simulink model "backups"  (R2024a)
settings: Solver=VariableStepAuto  StartTime=0.0  StopTime=10.0  RelTol=1e-3
values from neighbouring files (symbols this model uses):
  AttKd_x = inp(4,2).Var2    [SFF_Simulator_Entradas.m]
  AttKd_y = inp(5,2).Var2    [SFF_Simulator_Entradas.m]
  AttKd_z = inp(6,2).Var2    [SFF_Simulator_Entradas.m]
  AttKp_x = inp(1,2).Var2    [SFF_Simulator_Entradas.m]
  AttKp_y = inp(2,2).Var2    [SFF_Simulator_Entradas.m]
  AttKp_z = inp(3,2).Var2    [SFF_Simulator_Entradas.m]
  B = inp(8,2).Var2    [SFF_Simulator_Entradas.m]
  beta = inp(2,2).Var2    [SFF_Simulator_Entradas.m]
  Cd1 = inp(4,2).Var2    [SFF_Simulator_Entradas.m]
  cdgps = inp(1,2).Var2    [SFF_Simulator_Entradas.m]
  estrelas = inp(4,2).Var2    [SFF_Simulator_Entradas.m]
  estrelas_bias = inp(6,2).Var2    [SFF_Simulator_Entradas.m]
  estrelas_ruido = inp(5,2).Var2    [SFF_Simulator_Entradas.m]
  Fn = inp(2,2).Var2    [SFF_Simulator_Entradas.m]
  gps_bias = inp(3,2).Var2    [SFF_Simulator_Entradas.m]
  gps_ruido = inp(2,2).Var2    [SFF_Simulator_Entradas.m]
  Iw = inp(7,2).Var2    [SFF_Simulator_Entradas.m]
  Ixx = inp(7,2).Var2    [SFF_Simulator_Entradas.m]
  Iyy = inp(8,2).Var2    [SFF_Simulator_Entradas.m]
  Izz = inp(9,2).Var2    [SFF_Simulator_Entradas.m]
  Km = inp(3,2).Var2    [SFF_Simulator_Entradas.m]
  Kv = inp(9,2).Var2    [SFF_Simulator_Entradas.m]
  L1 = inp(5,2).Var2    [SFF_Simulator_Entradas.m]
  limCorrente = inp(4,2).Var2    [SFF_Simulator_Entradas.m]
  limVolt = inp(5,2).Var2    [SFF_Simulator_Entradas.m]
  m1 = inp(6,2).Var2    [SFF_Simulator_Entradas.m]
  magne = inp(10,2).Var2    [SFF_Simulator_Entradas.m]
  magne_bias = inp(12,2).Var2    [SFF_Simulator_Entradas.m]
  magne_ruido = inp(11,2).Var2    [SFF_Simulator_Entradas.m]
  man = inp(1,2).Var2    [SFF_Simulator_Entradas.m]
  OrbKd_x = inp(3,2).Var2    [SFF_Simulator_Entradas.m]
  OrbKd_y = inp(6,2).Var2    [SFF_Simulator_Entradas.m]
  OrbKd_z = inp(9,2).Var2    [SFF_Simulator_Entradas.m]
  OrbKi_x = inp(2,2).Var2    [SFF_Simulator_Entradas.m]
  OrbKi_y = inp(5,2).Var2    [SFF_Simulator_Entradas.m]
  OrbKi_z = inp(8,2).Var2    [SFF_Simulator_Entradas.m]
  OrbKp_x = inp(1,2).Var2    [SFF_Simulator_Entradas.m]
  OrbKp_y = inp(4,2).Var2    [SFF_Simulator_Entradas.m]
  OrbKp_z = inp(7,2).Var2    [SFF_Simulator_Entradas.m]
  propForcaAtivo = inp(1,2).Var2    [SFF_Simulator_Entradas.m]
  Rm = inp(6,2).Var2    [SFF_Simulator_Entradas.m]
  rodaAtivo = inp(1,2).Var2    [SFF_Simulator_Entradas.m]
  RodKi = inp(1,2).Var2    [SFF_Simulator_Entradas.m]
  sat_torquerod = inp(14,2).Var2    [SFF_Simulator_Entradas.m]
  torqrodAtivo = inp(1,2).Var2    [SFF_Simulator_Entradas.m]
undefined symbols (not defined in the file or in its folder): IAU, J2, mi, omega_E, propMomentoAtivo, Re, sat_rodareacao, WMM2020
libraries: dspsrcs4 x19, aerolibtransform2 x2, aerolibgravity2 x2, simulink x1
(part 1 of 4)
settings Model: VariantFading=off  Creator=rodri  LastModifiedBy=rodri

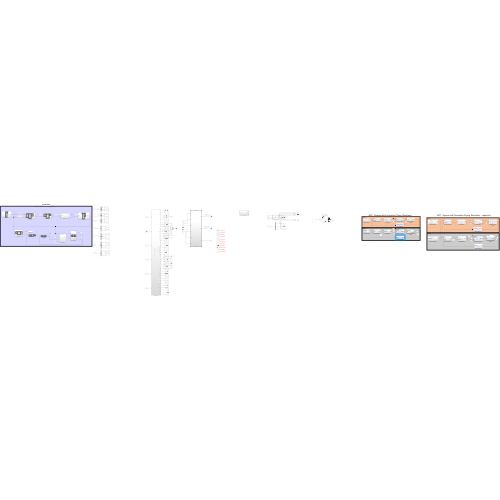
[thumbnail: Simulink's stored preview of the top-level diagram]
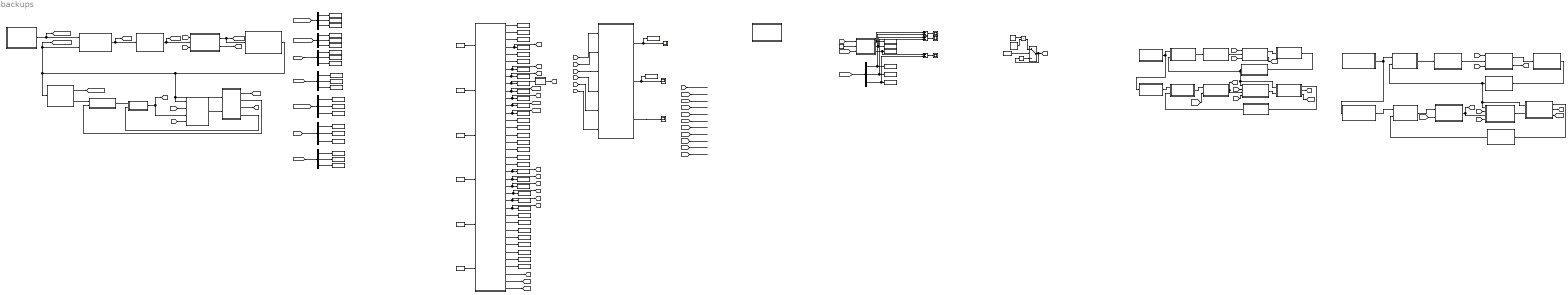
== system backups ==
  note: 13/04/2024
  note: Spacecraft Formation Flying Simulator
  note: Atitude
  note: SFF - Spacecraft Formation Flying Simulator
  note: Órbita
  note: Órbita
  note: SFF - Spacecraft Formation Flying Simulator - reduzido
  note: Atitude
  Atuadores Orbital : Subsystem
  Atuadores Orbital1 : Subsystem
  Atuadores de Atitude : Subsystem
  Atuadores de Atitude1 : Subsystem
  Bus Selector : BusSelector  OutputSignals=x_ref,y_ref,z_ref
  Bus Selector1 : BusSelector  OutputSignals=x,y,z
  Bus Selector2 : BusSelector  OutputSignals=erro_x,erro_y,erro_z
  Bus Selector3 : BusSelector  OutputSignals=phi_ref,theta_ref,psi_ref
  Bus Selector4 : BusSelector  OutputSignals=phi,theta,psi
  Constant : Constant  Value=Fn  SampleTime=-1
  Constant1 : Constant  Value=m1  SampleTime=-1
  Constant33 : Constant  Value=0
  Constant43 : Constant  Value=m1
  Constant45 : Constant  Value=0
  Constant46 : Constant  Value=0
  Constant48 : Constant  Value=Cd1
  Constant57 : Constant  Value=L1
  Controle Atitude : Subsystem
  Controle Atitude1 : Subsystem
  Controle Orbital : Subsystem
  Controle Orbital1 : Subsystem
  ControleAtitude1 : Subsystem
  Demux : Demux  Outputs=3
  Demux1 : Demux  Outputs=3
  Demux2 : Demux  Outputs=3
  Detect Decrease : simulink/Logic and Bit Operations/Detect Decrease  vinit=0.0  OutDataTypeStr=boolean
  Dinâmica Cinemática Atitude : Subsystem
  Dinâmica Cinemática Atitude1 : Subsystem
  Dinâmica Cinemática Orbital : Subsystem
  Dinâmica Cinemática Orbital1 : Subsystem
  DinâmicaCinematicaOrbital : Subsystem
  Erros Posição Orbital : Subsystem
  Erros Posição Orbital1 : Subsystem
  Erros Quatérnions : Subsystem
  Erros Quatérnions1 : Subsystem
  Guiamento Atitude : Subsystem
  Guiamento Atitude1 : Subsystem
  Guiamento Orbital : Subsystem
  Guiamento Orbital1 : Subsystem
  GuiamentoAtitude : Subsystem
  GuiamentoOrbital : Subsystem
  GuiamentoOrbital1 : Subsystem
  Memory1 : Memory  InitialCondition=Fn  InheritSampleTime=on
  Minus : Sum  Inputs=+-
  Minus1 : Sum  Inputs=+-
  Minus2 : Sum  Inputs=+-
  Product : Product
  Random Source2 : dspsrcs4/Random Source  SrcType=Uniform  MinVal=1-5/100  MaxVal=1+5/100  MeanVal=0  VarVal=1  RepMode=Not repeatable  rawSeed=1  IsInherit=off  SampTime=step_modelo  SampFrame=1  OutComplex=Real  DataType=double  SimulateUsing=Code generation
  Scope{1..6} (6 alike) : Scope
  Sensores Atitude : Subsystem
  Sensores Atitude1 : Subsystem
  Sensores Orbital : Subsystem
  Sensores Orbital1 : Subsystem
  Subsystem1 : ModelReference  ModelNameDialog=GuiamentoAtitude  ModelReferenceVersion=3.9
  Switch1 : Switch  Criteria=u2 > Threshold  SaturateOnIntegerOverflow=off  InputSameDT=off
  To Workspace : ToWorkspace  VariableName=x_ref  SaveFormat=Timeseries  SampleTime=-1
  To Workspace1 : ToWorkspace  VariableName=y_ref  SaveFormat=Timeseries  SampleTime=-1
  To Workspace10 : ToWorkspace  VariableName=uy  SaveFormat=Timeseries  SampleTime=-1
  To Workspace11 : ToWorkspace  VariableName=uz  SaveFormat=Timeseries  SampleTime=-1
  To Workspace12 : ToWorkspace  VariableName=phi_ref  SaveFormat=Timeseries  SampleTime=-1
  To Workspace13 : ToWorkspace  VariableName=theta_ref  SaveFormat=Timeseries  SampleTime=-1
  To Workspace14 : ToWorkspace  VariableName=psi_ref  SaveFormat=Timeseries  SampleTime=-1
  To Workspace15 : ToWorkspace  VariableName=phi  SaveFormat=Timeseries  SampleTime=-1
  To Workspace16 : ToWorkspace  VariableName=theta  SaveFormat=Timeseries  SampleTime=-1
  To Workspace17 : ToWorkspace  VariableName=psi  SaveFormat=Timeseries  SampleTime=-1
  To Workspace18 : ToWorkspace  VariableName=acely  SaveFormat=Timeseries  SampleTime=-1
  To Workspace19 : ToWorkspace  VariableName=acelz  SaveFormat=Timeseries  SampleTime=-1
  To Workspace2 : ToWorkspace  VariableName=z_ref  SaveFormat=Timeseries  SampleTime=-1
  To Workspace20 : ToWorkspace  VariableName=acelx  SaveFormat=Timeseries  SampleTime=-1
  To Workspace21 : ToWorkspace  VariableName=phi_ref1  SaveFormat=Timeseries  SampleTime=-1
  To Workspace22 : ToWorkspace  VariableName=theta_ref1  SaveFormat=Timeseries  SampleTime=-1
  To Workspace23 : ToWorkspace  VariableName=Fy_b_pro  SampleTime=-1
      settings: Save2DSignal=2-D array (concatenate along first dimension)
  To Workspace24 : ToWorkspace  VariableName=Fz_b_pro  SampleTime=-1
      settings: Save2DSignal=2-D array (concatenate along first dimension)
  To Workspace25 : ToWorkspace  VariableName=Fx_b_pro  SampleTime=-1
      settings: Save2DSignal=2-D array (concatenate along first dimension)
  To Workspace27 : ToWorkspace  VariableName=Fy_b_dem  SampleTime=-1
      settings: Save2DSignal=2-D array (concatenate along first dimension)
  To Workspace28 : ToWorkspace  VariableName=Fz_b_dem  SampleTime=-1
      settings: Save2DSignal=2-D array (concatenate along first dimension)
  To Workspace29 : ToWorkspace  VariableName=Fx_b_dem  SampleTime=-1
      settings: Save2DSignal=2-D array (concatenate along first dimension)
  To Workspace3 : ToWorkspace  VariableName=x  SaveFormat=Timeseries  SampleTime=-1
  To Workspace34 : ToWorkspace  VariableName=x_dotdot  SaveFormat=Timeseries  SampleTime=-1
  To Workspace35 : ToWorkspace  VariableName=y_dotdot  SaveFormat=Timeseries  SampleTime=-1
  To Workspace36 : ToWorkspace  VariableName=ohm0  SaveFormat=Timeseries  SampleTime=-1
  To Workspace37 : ToWorkspace  VariableName=omega_x  SaveFormat=Timeseries  SampleTime=-1
  To Workspace38 : ToWorkspace  VariableName=omega_z  SaveFormat=Timeseries  SampleTime=-1
  To Workspace39 : ToWorkspace  VariableName=dx0  SaveFormat=Timeseries  SampleTime=-1
  To Workspace4 : ToWorkspace  VariableName=y  SaveFormat=Timeseries  SampleTime=-1
  To Workspace40 : ToWorkspace  VariableName=dy0  SaveFormat=Timeseries  SampleTime=-1
  To Workspace41 : ToWorkspace  VariableName=dz0  SaveFormat=Timeseries  SampleTime=-1
  To Workspace47 : ToWorkspace  VariableName=delta_Dx  SaveFormat=Timeseries  SampleTime=-1
  To Workspace48 : ToWorkspace  VariableName=delta_Dy  SaveFormat=Timeseries  SampleTime=-1
  To Workspace49 : ToWorkspace  VariableName=delta_Dz  SaveFormat=Timeseries  SampleTime=-1
  To Workspace5 : ToWorkspace  VariableName=z  SaveFormat=Timeseries  SampleTime=-1
  To Workspace50 : ToWorkspace  VariableName=rho_a0  SaveFormat=Timeseries  SampleTime=-1
  To Workspace51 : ToWorkspace  VariableName=z_dotdot  SaveFormat=Timeseries  SampleTime=-1
  To Workspace52 : ToWorkspace  VariableName=x1  SaveFormat=Timeseries  SampleTime=-1
  To Workspace53 : ToWorkspace  VariableName=x_dot  SaveFormat=Timeseries  SampleTime=-1
  To Workspace54 : ToWorkspace  VariableName=y1  SaveFormat=Timeseries  SampleTime=-1
  To Workspace55 : ToWorkspace  VariableName=y_dot  SaveFormat=Timeseries  SampleTime=-1
  To Workspace56 : ToWorkspace  VariableName=z1  SaveFormat=Timeseries  SampleTime=-1
  To Workspace57 : ToWorkspace  VariableName=z_dot  SaveFormat=Timeseries  SampleTime=-1
  To Workspace58 : ToWorkspace  VariableName=rho_a1  SaveFormat=Timeseries  SampleTime=-1
  To Workspace59 : ToWorkspace  VariableName=r0_dotdot  SaveFormat=Timeseries  SampleTime=-1
  To Workspace6 : ToWorkspace  VariableName=erro_x  SaveFormat=Timeseries  SampleTime=-1
  To Workspace60 : ToWorkspace  VariableName=omega_z_dot  SaveFormat=Timeseries  SampleTime=-1
  To Workspace61 : ToWorkspace  VariableName=dx1  SaveFormat=Timeseries  SampleTime=-1
  To Workspace62 : ToWorkspace  VariableName=r0  SaveFormat=Timeseries  SampleTime=-1
  To Workspace63 : ToWorkspace  VariableName=dy1  SaveFormat=Timeseries  SampleTime=-1
  To Workspace64 : ToWorkspace  VariableName=dz1  SaveFormat=Timeseries  SampleTime=-1
  To Workspace65 : ToWorkspace  VariableName=omega_y_dot  SaveFormat=Timeseries  SampleTime=-1
  To Workspace66 : ToWorkspace  VariableName=omega_x_dot  SaveFormat=Timeseries  SampleTime=-1
  To Workspace67 : ToWorkspace  VariableName=h0  SaveFormat=Timeseries  SampleTime=-1
  To Workspace68 : ToWorkspace  VariableName=r1  SaveFormat=Timeseries  SampleTime=-1
  To Workspace69 : ToWorkspace  VariableName=r0_dot  SaveFormat=Timeseries  SampleTime=-1
  To Workspace7 : ToWorkspace  VariableName=erro_y  SaveFormat=Timeseries  SampleTime=-1
  To Workspace70 : ToWorkspace  VariableName=i0  SaveFormat=Timeseries  SampleTime=-1
  To Workspace71 : ToWorkspace  VariableName=theta0  SaveFormat=Timeseries  SampleTime=-1
  To Workspace72 : ToWorkspace  VariableName=theta0_dot  SaveFormat=Timeseries  SampleTime=-1
  To Workspace8 : ToWorkspace  VariableName=erro_z  SaveFormat=Timeseries  SampleTime=-1
  To Workspace9 : ToWorkspace  VariableName=ux  SaveFormat=Timeseries  SampleTime=-1
  atuadoresAtitude : Subsystem
  atuadoresOrbital : Subsystem
  atuadoresOrbital1 : Subsystem
  controleOrbital : Subsystem
  dinamicaCinematicaAtitude1 : Subsystem
  errosAngAtitude1 : Subsystem
  errosPosVelOrbital : Subsystem
  forçasSistCorpoSeg1 : MATLAB Function  TreatAsAtomicUnit=on
  wrapTo2Pi1 : MATLAB Function  TreatAsAtomicUnit=on
  wires:
  Bus Selector4/3 -> To Workspace17/1  "<psi>"
  Bus Selector4/2 -> To Workspace16/1  "<theta>"
  ControleAtitude1/1(Mts) -> atuadoresAtitude/3(Mts), [Mts]
  Demux/3 -> To Workspace11/1
  atuadoresAtitude/1(MtsReal) -> dinamicaCinematicaAtitude1/2(Mts)
  [atitude] -> Bus Selector4/1
  [Mts] -> atuadoresOrbital/3(Mts)
  Bus Selector4/1 -> To Workspace15/1  "<phi>"
  Bus Selector1/2 -> To Workspace4/1  "<y>"
  dinamicaCinematicaAtitude1/4(omega_rel) -> ControleAtitude1/2(omega_rel)
  [MtsProp] -> atuadoresAtitude/2(MtsProp)
  Bus Selector1/3 -> To Workspace5/1  "<z>"
  [guiamentoAtitude] -> Bus Selector3/1
  Demux1/3 -> To Workspace19/1
  Demux1/1 -> To Workspace20/1
  Bus Selector/2 -> To Workspace1/1  "<y_ref>"
  DinâmicaCinematicaOrbital/1(dinamicaCinematicaOrbital) -> atuadoresAtitude/1(dinamicaCinematicaOrbital), dinamicaCinematicaAtitude1/1(dinamicaCinematicaOrbital), errosPosVelOrbital/2(dinamicaCinematicaOrbital), [dinamicaCinematicaOrbital], GuiamentoAtitude/1(dinamicaCinematicaOrbital)
  [A_q] -> atuadoresAtitude/4(A_q)
  [acelControle] -> Demux1/1
  Bus Selector3/3 -> To Workspace14/1  "<psi_ref>"
  Bus Selector2/2 -> To Workspace7/1  "<erro_y>"
  [controleOrbital] -> Demux/1
  dinamicaCinematicaAtitude1/2(q_rel) -> errosAngAtitude1/2(q_rel)
  GuiamentoAtitude/2(q_ref) -> errosAngAtitude1/1(q_ref)
  Demux1/2 -> To Workspace18/1
  atuadoresOrbital/1(acelControle) -> [acelControle], DinâmicaCinematicaOrbital/1(controleOrbital)
  Bus Selector1/1 -> To Workspace3/1  "<x>"
  [dinamicaCinematicaOrbital] -> Bus Selector1/1
  Bus Selector2/3 -> To Workspace8/1  "<erro_z>"
  dinamicaCinematicaAtitude1/1(euler) -> [atitude]
  errosAngAtitude1/1(q_erro) -> ControleAtitude1/1(q_erro)
  [errosOrbital] -> Bus Selector2/1
  controleOrbital/1(controleOrbital) -> atuadoresOrbital/2(controleOrbital), [controleOrbital]
  Demux/1 -> To Workspace9/1
  Bus Selector2/1 -> To Workspace6/1  "<erro_x>"
  GuiamentoAtitude/1(eulerRef) -> [guiamentoAtitude]
  [A_q] -> atuadoresOrbital/1(A_q)
  Demux/2 -> To Workspace10/1
  Bus Selector3/2 -> To Workspace13/1  "<theta_ref>"
  Bus Selector/3 -> To Workspace2/1  "<z_ref>"
  errosPosVelOrbital/1(errosOrbital) -> controleOrbital/1(errosOrbital), [errosOrbital]
  Bus Selector3/1 -> To Workspace12/1  "<phi_ref>"
  Bus Selector/1 -> To Workspace/1  "<x_ref>"
  atuadoresOrbital/2(MtsProp) -> [MtsProp]
  [guiamentoOrbital] -> Bus Selector/1
  dinamicaCinematicaAtitude1/3(A_q) -> [A_q]
  GuiamentoOrbital/1(guiamentoOrbital) -> [guiamentoOrbital], errosPosVelOrbital/1(guiamentoOrbital)
  [r0] -> ?
  [theta0_dot] -> ?
  [r0_dot] -> ?
  [i0_dot] -> ?
  [omega_z] -> ?
  [omega_x] -> ?
  [omega_y] -> ?
  [ohm0] -> ?
  [ohm0_dot] -> ?
  GuiamentoOrbital1/28(r0_dotdot) -> To Workspace59/1
  GuiamentoOrbital1/30(dx1) -> To Workspace61/1
  GuiamentoOrbital1/35(i0_dot) -> [i0_dot]
  [theta0] -> ?
  GuiamentoOrbital1/21(x) -> To Workspace52/1, [x]
  GuiamentoOrbital1/15(dy0) -> To Workspace40/1
  GuiamentoOrbital1/34(omega_x_dot) -> To Workspace66/1
  GuiamentoOrbital1/11(ohm0) -> [ohm0], To Workspace36/1
  GuiamentoOrbital1/9(theta0) -> To Workspace71/1, wrapTo2Pi1/1(u)
  GuiamentoOrbital1/12(omega_x) -> To Workspace37/1, [omega_x]
  [i0] -> ?
  GuiamentoOrbital1/32(dz1) -> To Workspace64/1
  GuiamentoOrbital1/8(i0) -> [i0], To Workspace70/1
  GuiamentoOrbital1/36(ohm0_dot) -> [ohm0_dot]
  GuiamentoOrbital1/1(x_dotdot) -> To Workspace34/1
  Constant48/1 -> GuiamentoOrbital1/2(Cd1)
  GuiamentoOrbital1/22(x_dot) -> To Workspace53/1, [x_dot]
  GuiamentoOrbital1/13(omega_z) -> [omega_z], To Workspace38/1
  GuiamentoOrbital1/19(delta_Dz) -> To Workspace49/1
  GuiamentoOrbital1/20(rho_a0) -> To Workspace50/1
  Constant43/1 -> GuiamentoOrbital1/1(m1)
  GuiamentoOrbital1/10(theta0_dot) -> [theta0_dot], To Workspace72/1
  Subsystem1/2 -> Scope2/1, To Workspace22/1
  Constant33/1 -> GuiamentoOrbital1/4(ux)
  GuiamentoOrbital1/7(r0_dot) -> To Workspace69/1, [r0_dot]
  GuiamentoOrbital1/26(z_dot) -> [z_dot], To Workspace57/1
  [y_dot] -> Subsystem1/5
  GuiamentoOrbital1/3(z_dotdot) -> To Workspace51/1
  GuiamentoOrbital1/31(dy1) -> To Workspace63/1
  wrapTo2Pi1/1(y) -> [theta0]
  GuiamentoOrbital1/17(delta_Dx) -> To Workspace47/1
  GuiamentoOrbital1/2(y_dotdot) -> To Workspace35/1
  GuiamentoOrbital1/23(y) -> To Workspace54/1, [y]
  GuiamentoOrbital1/5(h0) -> To Workspace67/1
  Subsystem1/1 -> To Workspace21/1, Scope1/1
  GuiamentoOrbital1/27(rho_a1) -> To Workspace58/1
  GuiamentoOrbital1/29(omega_z_dot) -> To Workspace60/1
  GuiamentoOrbital1/6(r1) -> To Workspace68/1
  GuiamentoOrbital1/37(omega_y) -> [omega_y]
  GuiamentoOrbital1/18(delta_Dy) -> To Workspace48/1
  GuiamentoOrbital1/25(z) -> To Workspace56/1, [z]
  [x_dot] -> Subsystem1/4
  GuiamentoOrbital1/14(dx0) -> To Workspace39/1
  GuiamentoOrbital1/33(omega_y_dot) -> To Workspace65/1
  Constant45/1 -> GuiamentoOrbital1/5(uy)
  Constant46/1 -> GuiamentoOrbital1/6(uz)
  Constant57/1 -> GuiamentoOrbital1/3(l1)
  [x] -> Subsystem1/1
  [z] -> Subsystem1/3
  GuiamentoOrbital1/24(y_dot) -> To Workspace55/1, [y_dot]
  Subsystem1/3 -> Scope3/1
  [z_dot] -> Subsystem1/6
  GuiamentoOrbital1/16(dz0) -> To Workspace41/1
  GuiamentoOrbital1/4(r0) -> To Workspace62/1, [r0]
  [y] -> Subsystem1/2
  Minus2/1 -> Scope6/1
  [A_q] -> forçasSistCorpoSeg1/1(A_q)
  [controleOrbital] -> forçasSistCorpoSeg1/3(controleOrbital)
  forçasSistCorpoSeg1/1(Fx_b) -> To Workspace29/1, Minus/1
  forçasSistCorpoSeg1/2(Fy_b) -> To Workspace27/1, Minus1/1
  Demux2/3 -> To Workspace24/1, Minus2/2
  forçasSistCorpoSeg1/3(Fz_b) -> To Workspace28/1, Minus2/1
  Minus/1 -> Scope4/1
  [forcasProp] -> Demux2/1
  Constant1/1 -> forçasSistCorpoSeg1/2(m1)
  Minus1/1 -> Scope5/1
  Demux2/2 -> To Workspace23/1, Minus1/2
  Demux2/1 -> To Workspace25/1, Minus/2
  ? -> Detect Decrease/1  "PWM"
  Constant/1 -> Product/1
  Detect Decrease/1 -> Switch1/2
  Memory1/1 -> Switch1/3
  Product/1 -> Switch1/1
  Switch1/1 -> [F_real], Memory1/1
  Random Source2/1 -> Product/2
  Controle Atitude/1(Mts) -> Atuadores de Atitude/3(Mts), [Mts]
  Atuadores de Atitude/1(MtsReal) -> Dinâmica Cinemática Atitude/2(Mts)
  [omega_rel] -> Controle Atitude/2(omega_rel)
  [A_q] -> Atuadores de Atitude/4(A_q)
  [Mts] -> Atuadores Orbital/3(Mts)
  Atuadores Orbital/2(MtsProp) -> [MtsProp]
  Controle Orbital/1(conOrb) -> Atuadores Orbital/2(conOrb)
  Dinâmica Cinemática Atitude/3(omega_rel) -> [omega_rel]
  Erros Quatérnions/1(q_erro) -> Controle Atitude/1(q_erro)
  Sensores Orbital/1(dinCinOrbOut) -> Dinâmica Cinemática Atitude/1(dinCinOrb), Atuadores de Atitude/1(dinCinOrb), Erros Posição Orbital/2(dinCinOrb)
  Guiamento Orbital/1(guiOrb) -> Guiamento Atitude/1(dinCinOrb), Erros Posição Orbital/1(guiOrb)
  Dinâmica Cinemática Atitude/1(q_rel) -> Sensores Atitude/1(qRelIn)
  Dinâmica Cinemática Atitude/2(A_q) -> [A_q]
  Dinâmica Cinemática Orbital/1(dinCinOrb) -> Sensores Orbital/1(dinCinOrbIn)
  [A_q] -> Atuadores Orbital/1(A_q)
  Guiamento Atitude/1(q_ref) -> Erros Quatérnions/1(q_ref)
  Erros Posição Orbital/1(errOrb) -> Controle Orbital/1(errOrb)
  [MtsProp] -> Atuadores de Atitude/2(MtsProp)
  Atuadores Orbital/1(aceCon) -> Dinâmica Cinemática Orbital/1(conOrb)
  Sensores Atitude/1(qRelOut) -> Erros Quatérnions/2(q_rel)
  Sensores Orbital1/1(dinCinOrbSen) -> Dinâmica Cinemática Atitude1/1(dinCinOrb), Atuadores de Atitude1/1(dinCinOrb), Erros Posição Orbital1/2(dinCinOrb)
  Erros Posição Orbital1/1(errOrb) -> Controle Orbital1/1(errOrb)
  Guiamento Orbital1/1(guiOrb) -> Guiamento Atitude1/1(dinCinOrb), Erros Posição Orbital1/1(guiOrb)
  Dinâmica Cinemática Atitude1/1(q_rel) -> Sensores Atitude1/1(qRel)
  Sensores Atitude1/1(qRelSen) -> Erros Quatérnions1/2(q_rel)
  Atuadores Orbital1/1(aceCon) -> Dinâmica Cinemática Orbital1/1(conOrb)
  [A_q] -> Atuadores Orbital1/1(A_q)
  Dinâmica Cinemática Atitude1/3(omega_rel) -> [omega_rel]
  [omega_rel] -> Controle Atitude1/2(omega_rel)
  Atuadores Orbital1/2(MtsProp) -> [MtsProp]
  Erros Quatérnions1/1(q_erro) -> Controle Atitude1/1(q_erro)
  Dinâmica Cinemática Orbital1/1(dinCinOrb) -> Sensores Orbital1/1(dinCinOrb)
  [A_q] -> Atuadores de Atitude1/4(A_q)
  Controle Atitude1/1(Mts) -> Atuadores de Atitude1/3(Mts), [Mts]
  Atuadores de Atitude1/1(MtsReal) -> Dinâmica Cinemática Atitude1/2(Mts)
  Dinâmica Cinemática Atitude1/2(A_q) -> [A_q]
  Controle Orbital1/1(conOrb) -> Atuadores Orbital1/2(conOrb)
  Guiamento Atitude1/1(q_ref) -> Erros Quatérnions1/1(q_ref)
  [Mts] -> Atuadores Orbital1/3(Mts)
  [MtsProp] -> Atuadores de Atitude1/2(MtsProp)

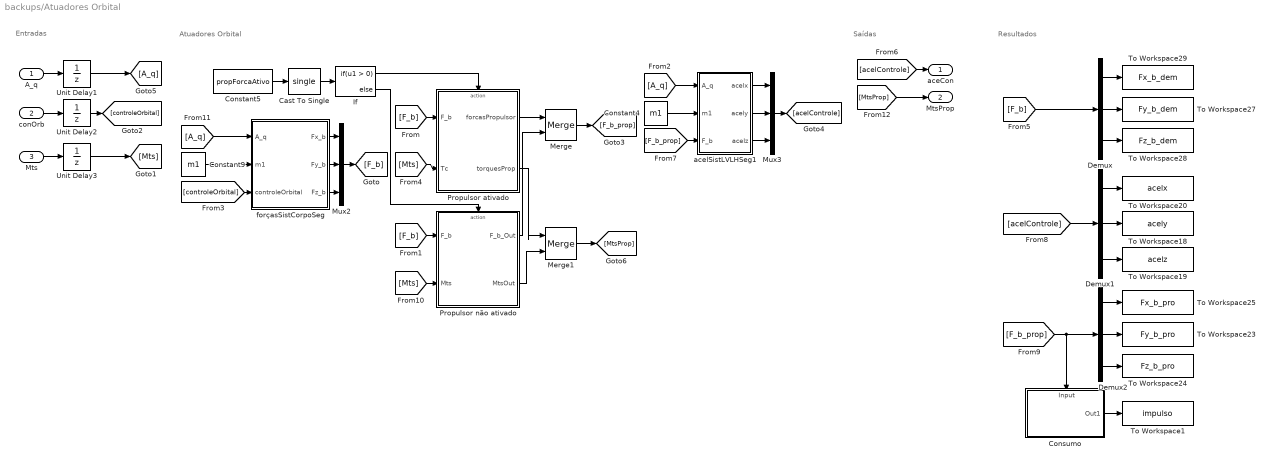
== system backups/Atuadores Orbital ==
  note: Resultados
  note: Entradas
  note: Saídas
  note: Atuadores Orbital
  A_q : Inport
  conOrb : Inport  Port=2
  Mts : Inport  Port=3
  Cast To Single : DataTypeConversion  OutDataTypeStr=single  SaturateOnIntegerOverflow=off  RndMeth=Floor
  Constant4 : Constant  Value=m1  SampleTime=-1
  Constant5 : Constant  Value=propForcaAtivo  SampleTime=-1
  Constant9 : Constant  Value=m1  SampleTime=-1
  Consumo : Subsystem
      settings: PortSchema="{\"entries\":[{\"content\":{\"sides\":[{\"content\":{},\"type\":\"ConnectorPlacement.EquallySpacedRectSide\",\"uuid\":\"7adfb598-cfd3-455e-a32c-0f282c9a4562\"},{\"content\":{\"connectorIds\":[\"Out1\"],\"side\":\"RIGHT\"},\"type\":\"ConnectorPlacement.EquallySpacedRectSide\",\"uuid\":\"983f0880-1b1d-4863-83b8-6f46272dfc63\"},{\"content\":{\"connectorIds\":[\"In1\"],\"side\":\"TOP\"},\"type\":\"ConnectorPlacement.EquallySpacedRectSide\",\"uuid\":\"1e4b7baa-07be-492c-ad2b-c1f0c72f4a8d\"}]},\"type\":\"ConnectorPlacement.EquallySpacedConnector\",\"uuid\":\"1ca021a5-bfd9-4f0e-bb93-1261a452b994\"}],\"packageUris\":[\"http://schema.mathworks.com/mf0/Connector/R2020b\"],\"version\":\"1.0\"}"
  Demux : Demux  Outputs=3
  Demux1 : Demux  Outputs=3
  Demux2 : Demux  Outputs=3
  If : If
  Merge : Merge
  Merge1 : Merge
  Mux2 : Mux  Inputs=3
  Mux3 : Mux  Inputs=3
  Propulsor ativado : Subsystem  TreatAsAtomicUnit=on
  Propulsor não ativado : Subsystem  TreatAsAtomicUnit=on
  To Workspace1 : ToWorkspace  VariableName=impulso  SampleTime=-1
      settings: Save2DSignal=2-D array (concatenate along first dimension)
  To Workspace18 : ToWorkspace  VariableName=acely  SampleTime=-1
      settings: Save2DSignal=2-D array (concatenate along first dimension)
  To Workspace19 : ToWorkspace  VariableName=acelz  SampleTime=-1
      settings: Save2DSignal=2-D array (concatenate along first dimension)
  To Workspace20 : ToWorkspace  VariableName=acelx  SampleTime=-1
      settings: Save2DSignal=2-D array (concatenate along first dimension)
  To Workspace23 : ToWorkspace  VariableName=Fy_b_pro  SampleTime=-1
      settings: Save2DSignal=2-D array (concatenate along first dimension)
  To Workspace24 : ToWorkspace  VariableName=Fz_b_pro  SampleTime=-1
      settings: Save2DSignal=2-D array (concatenate along first dimension)
  To Workspace25 : ToWorkspace  VariableName=Fx_b_pro  SampleTime=-1
      settings: Save2DSignal=2-D array (concatenate along first dimension)
  To Workspace27 : ToWorkspace  VariableName=Fy_b_dem  SampleTime=-1
      settings: Save2DSignal=2-D array (concatenate along first dimension)
  To Workspace28 : ToWorkspace  VariableName=Fz_b_dem  SampleTime=-1
      settings: Save2DSignal=2-D array (concatenate along first dimension)
  To Workspace29 : ToWorkspace  VariableName=Fx_b_dem  SampleTime=-1
      settings: Save2DSignal=2-D array (concatenate along first dimension)
  Unit Delay1 : UnitDelay  SampleTime=-1  HasFrameUpgradeWarning=on
  Unit Delay2 : UnitDelay  SampleTime=-1  HasFrameUpgradeWarning=on
  Unit Delay3 : UnitDelay  SampleTime=-1  HasFrameUpgradeWarning=on
  acelSistLVLHSeg1 : MATLAB Function  TreatAsAtomicUnit=on
  forçasSistCorpoSeg : MATLAB Function  TreatAsAtomicUnit=on
  aceCon : Outport
  MtsProp : Outport  Port=2
  wires:
  Demux1/3 -> To Workspace19/1
  Demux1/1 -> To Workspace20/1
  Demux1/2 -> To Workspace18/1
  [acelControle] -> Demux1/1
  Consumo/1(Out1) -> To Workspace1/1
  Demux/1 -> To Workspace29/1
  Demux/2 -> To Workspace27/1
  Demux/3 -> To Workspace28/1
  [F_b] -> Demux/1
  Demux2/1 -> To Workspace25/1
  [F_b_prop] -> Demux2/1, Consumo/1(Input)
  Demux2/2 -> To Workspace23/1
  Demux2/3 -> To Workspace24/1
  [A_q] -> acelSistLVLHSeg1/1(A_q)
  [acelControle] -> aceCon/1
  [F_b_prop] -> acelSistLVLHSeg1/3(F_b)
  [MtsProp] -> MtsProp/1
  Constant4/1 -> acelSistLVLHSeg1/2(m1)
  Propulsor ativado/2(torquesProp) -> Merge1/1
  Merge/1 -> [F_b_prop]
  forçasSistCorpoSeg/3(Fz_b) -> Mux2/3
  Unit Delay1/1 -> [A_q]
  Merge1/1 -> [MtsProp]
  forçasSistCorpoSeg/1(Fx_b) -> Mux2/1
  If/2 -> Propulsor não ativado/Action
  If/1 -> Propulsor ativado/Action
  Unit Delay2/1 -> [controleOrbital]
  [Mts] -> Propulsor não ativado/2(Mts)
  [A_q] -> forçasSistCorpoSeg/1(A_q)
  Constant9/1 -> forçasSistCorpoSeg/2(m1)
  [controleOrbital] -> forçasSistCorpoSeg/3(controleOrbital)
  [Mts] -> Propulsor ativado/2(Tc)
  acelSistLVLHSeg1/1(acelx) -> Mux3/1
  Mux3/1 -> [acelControle]
  acelSistLVLHSeg1/3(acelz) -> Mux3/3
  acelSistLVLHSeg1/2(acely) -> Mux3/2
  forçasSistCorpoSeg/2(Fy_b) -> Mux2/2
  Propulsor ativado/1(forcasPropulsor) -> Merge/1
  Cast To Single/1 -> If/1
  Mux2/1 -> [F_b]
  Mts/1 -> Unit Delay3/1
  [F_b] -> Propulsor não ativado/1(F_b)
  conOrb/1 -> Unit Delay2/1
  Propulsor não ativado/1(F_b_Out) -> Merge/2
  Unit Delay3/1 -> [Mts]
  Constant5/1 -> Cast To Single/1
  [F_b] -> Propulsor ativado/1(F_b)
  Propulsor não ativado/2(MtsOut) -> Merge1/2
  A_q/1 -> Unit Delay1/1

== system backups/Atuadores Orbital1 ==
  note: Saídas
  note: Resultados
  note: Atuadores Orbital
  note: Entradas
  A_q : Inport
  conOrb : Inport  Port=2
  Mts : Inport  Port=3
  Cast To Single : DataTypeConversion  OutDataTypeStr=single  SaturateOnIntegerOverflow=off  RndMeth=Floor
  Constant4 : Constant  Value=m1  SampleTime=-1
  Constant5 : Constant  Value=propForcaAtivo  SampleTime=-1
  Constant9 : Constant  Value=m1  SampleTime=-1
  Consumo : Subsystem
      settings: PortSchema="{\"entries\":[{\"content\":{\"sides\":[{\"content\":{},\"type\":\"ConnectorPlacement.EquallySpacedRectSide\",\"uuid\":\"7adfb598-cfd3-455e-a32c-0f282c9a4562\"},{\"content\":{\"connectorIds\":[\"Out1\"],\"side\":\"RIGHT\"},\"type\":\"ConnectorPlacement.EquallySpacedRectSide\",\"uuid\":\"983f0880-1b1d-4863-83b8-6f46272dfc63\"},{\"content\":{\"connectorIds\":[\"In1\"],\"side\":\"TOP\"},\"type\":\"ConnectorPlacement.EquallySpacedRectSide\",\"uuid\":\"1e4b7baa-07be-492c-ad2b-c1f0c72f4a8d\"}]},\"type\":\"ConnectorPlacement.EquallySpacedConnector\",\"uuid\":\"1ca021a5-bfd9-4f0e-bb93-1261a452b994\"}],\"packageUris\":[\"http://schema.mathworks.com/mf0/Connector/R2020b\"],\"version\":\"1.0\"}"
  If : If
  Merge : Merge
  Merge1 : Merge
  Mux2 : Mux  Inputs=3
  Mux3 : Mux  Inputs=3
  Propulsor ativado : Subsystem  TreatAsAtomicUnit=on
  Propulsor não ativado : Subsystem  TreatAsAtomicUnit=on
  To Workspace1 : ToWorkspace  VariableName=impulso  SampleTime=-1
      settings: Save2DSignal=2-D array (concatenate along first dimension)
  Unit Delay1 : UnitDelay  SampleTime=-1  HasFrameUpgradeWarning=on
  Unit Delay2 : UnitDelay  SampleTime=-1  HasFrameUpgradeWarning=on
  Unit Delay3 : UnitDelay  SampleTime=-1  HasFrameUpgradeWarning=on
  acelSistLVLHSeg1 : MATLAB Function  TreatAsAtomicUnit=on
  forçasSistCorpoSeg : MATLAB Function  TreatAsAtomicUnit=on
  aceCon : Outport
  MtsProp : Outport  Port=2
  wires:
  A_q/1 -> Unit Delay1/1
  conOrb/1 -> Unit Delay2/1
  Mts/1 -> Unit Delay3/1
  Constant5/1 -> Cast To Single/1
  Cast To Single/1 -> If/1
  If/1 -> Propulsor ativado/Action
  [Mts] -> Propulsor não ativado/2(Mts)
  [F_b] -> Propulsor não ativado/1(F_b)
  Propulsor não ativado/1(F_b_Out) -> Merge/2
  Propulsor ativado/1(forcasPropulsor) -> Merge/1
  Propulsor não ativado/2(MtsOut) -> Merge1/2
  Propulsor ativado/2(torquesProp) -> Merge1/1
  [F_b] -> Propulsor ativado/1(F_b)
  If/2 -> Propulsor não ativado/Action
  Unit Delay1/1 -> [A_q]
  Unit Delay2/1 -> [controleOrbital]
  Unit Delay3/1 -> [Mts]
  Mux2/1 -> [F_b]
  [A_q] -> forçasSistCorpoSeg/1(A_q)
  forçasSistCorpoSeg/3(Fz_b) -> Mux2/3
  Constant9/1 -> forçasSistCorpoSeg/2(m1)
  [controleOrbital] -> forçasSistCorpoSeg/3(controleOrbital)
  forçasSistCorpoSeg/2(Fy_b) -> Mux2/2
  forçasSistCorpoSeg/1(Fx_b) -> Mux2/1
  [Mts] -> Propulsor ativado/2(Tc)
  acelSistLVLHSeg1/3(acelz) -> Mux3/3
  Constant4/1 -> acelSistLVLHSeg1/2(m1)
  acelSistLVLHSeg1/1(acelx) -> Mux3/1
  [F_b_prop] -> acelSistLVLHSeg1/3(F_b)
  acelSistLVLHSeg1/2(acely) -> Mux3/2
  Mux3/1 -> [acelControle]
  [A_q] -> acelSistLVLHSeg1/1(A_q)
  Consumo/1(Out1) -> To Workspace1/1
  [acelControle] -> aceCon/1
  Merge/1 -> [F_b_prop]
  [F_b_prop] -> Consumo/1(Input)
  Merge1/1 -> [MtsProp]
  [MtsProp] -> MtsProp/1

== system backups/Atuadores de Atitude ==
  note: Entradas
  note: Atuadores Atitude
  note: Saídas
  dinCinOrb : Inport
  MtsProp : Inport  Port=2
  Mts : Inport  Port=3
  A_q : Inport  Port=4
  Atuador atitude ativado : Subsystem  TreatAsAtomicUnit=on
  Atuador atitude desativado : Subsystem  TreatAsAtomicUnit=on
  Cast To Single : DataTypeConversion  OutDataTypeStr=single  SaturateOnIntegerOverflow=off  RndMeth=Floor
  Constant4 : Constant  Value=rodaAtivo  SampleTime=-1
  Constant5 : Constant  Value=propForcaAtivo  SampleTime=-1
  Constant9 : Constant  Value=torqrodAtivo  SampleTime=-1
  If : If
  Logical Operator : Logic  Operator=OR  Inputs=3  AllPortsSameDT=off  OutDataTypeStr=boolean
  Merge : Merge
  MtsReal : Outport
  wires:
  Mts/1 -> [Mts]
  dinCinOrb/1 -> [dinCinOrb]
  MtsProp/1 -> [MtsProp]
  Merge/1 -> [MtsReal]
  If/1 -> Atuador atitude ativado/Action
  If/2 -> Atuador atitude desativado/Action
  Atuador atitude ativado/1(MtsReal) -> Merge/1
  Atuador atitude desativado/1(Out1) -> Merge/2
  [Mts] -> Atuador atitude desativado/1(In1)
  [MtsProp] -> Atuador atitude ativado/1(MtsProp)
  [Mts] -> Atuador atitude ativado/2(Mts)
  [dinCinOrb] -> Atuador atitude ativado/3(dinCinOrb)
  [A_q] -> Atuador atitude ativado/4(A_q)
  A_q/1 -> [A_q]
  [MtsReal] -> MtsReal/1
  Constant5/1 -> Logical Operator/1
  Logical Operator/1 -> Cast To Single/1
  Cast To Single/1 -> If/1
  Constant4/1 -> Logical Operator/2
  Constant9/1 -> Logical Operator/3

== system backups/Atuadores de Atitude1 ==
  note: Entradas
  note: Atuadores Atitude
  note: Saídas
  dinCinOrb : Inport
  MtsProp : Inport  Port=2
  Mts : Inport  Port=3
  A_q : Inport  Port=4
  Atuador atitude ativado : Subsystem  TreatAsAtomicUnit=on
  Atuador atitude desativado : Subsystem  TreatAsAtomicUnit=on
  Cast To Single : DataTypeConversion  OutDataTypeStr=single  SaturateOnIntegerOverflow=off  RndMeth=Floor
  Constant4 : Constant  Value=rodaAtivo  SampleTime=-1
  Constant5 : Constant  Value=propForcaAtivo  SampleTime=-1
  Constant9 : Constant  Value=torqrodAtivo  SampleTime=-1
  If : If
  Logical Operator : Logic  Operator=OR  Inputs=3  AllPortsSameDT=off  OutDataTypeStr=boolean
  Merge : Merge
  MtsReal : Outport
  wires:
  Mts/1 -> [Mts]
  dinCinOrb/1 -> [dinCinOrb]
  MtsProp/1 -> [MtsProp]
  Merge/1 -> [MtsReal]
  Logical Operator/1 -> Cast To Single/1
  Constant5/1 -> Logical Operator/1
  Constant4/1 -> Logical Operator/2
  Constant9/1 -> Logical Operator/3
  Cast To Single/1 -> If/1
  If/1 -> Atuador atitude ativado/Action
  If/2 -> Atuador atitude desativado/Action
  Atuador atitude ativado/1(MtsReal) -> Merge/1
  Atuador atitude desativado/1(Out1) -> Merge/2
  [Mts] -> Atuador atitude desativado/1(In1)
  [MtsProp] -> Atuador atitude ativado/1(MtsProp)
  [Mts] -> Atuador atitude ativado/2(Mts)
  [dinCinOrb] -> Atuador atitude ativado/3(dinCinOrb)
  [A_q] -> Atuador atitude ativado/4(A_q)
  A_q/1 -> [A_q]
  [MtsReal] -> MtsReal/1

== system backups/Controle Atitude ==
  note: Entradas
  note: Controle de Atitude
  note: Saídas
  note: Resultados
  q_erro : Inport
  omega_rel : Inport  Port=2
  Demux : Demux
  Demux1 : Demux  Outputs=3
  Demux3 : Demux  Outputs=3
  Gain1 : Gain  Gain=-1
  Kd1 : Gain  Gain=[AttKd_x AttKd_y AttKd_z]'
  Kp1 : Gain  Gain=[AttKp_x AttKp_y AttKp_z]'
  Mux : Mux  Inputs=3
  Sum3 : Sum  Inputs=|++
  Terminator : Terminator
  To Workspace24 : ToWorkspace  VariableName=Mts_x  SampleTime=-1
      settings: Save2DSignal=2-D array (concatenate along first dimension)
  To Workspace25 : ToWorkspace  VariableName=Mts_y  SampleTime=-1
      settings: Save2DSignal=2-D array (concatenate along first dimension)
  To Workspace26 : ToWorkspace  VariableName=Mts_z  SampleTime=-1
      settings: Save2DSignal=2-D array (concatenate along first dimension)
  Unit Delay : UnitDelay  SampleTime=-1  HasFrameUpgradeWarning=on
  Unit Delay1 : UnitDelay  SampleTime=-1  HasFrameUpgradeWarning=on
  Vector Concatenate1 : Concatenate  NumInputs=3  Mode=Multidimensional array
  Mts : Outport
  wires:
  [q_erro] -> Demux/1
  Mux/1 -> Kp1/1
  Demux/1 -> Mux/1
  Demux/2 -> Mux/2
  Demux/3 -> Mux/3
  Demux/4 -> Terminator/1
  [omega_rel] -> Kd1/1
  Kd1/1 -> Sum3/2
  Sum3/1 -> Demux1/1
  Demux1/1 -> Vector Concatenate1/1
  Demux1/2 -> Vector Concatenate1/2
  Demux1/3 -> Vector Concatenate1/3
  q_erro/1 -> Unit Delay/1
  omega_rel/1 -> Unit Delay1/1
  [Mts] -> Mts/1
  Vector Concatenate1/1 -> Gain1/1
  Gain1/1 -> [Mts]
  Kp1/1 -> Sum3/1
  Demux3/3 -> To Workspace26/1
  Demux3/2 -> To Workspace25/1
  Demux3/1 -> To Workspace24/1
  [Mts] -> Demux3/1
  Unit Delay/1 -> [q_erro]
  Unit Delay1/1 -> [omega_rel]

== system backups/Controle Atitude1 ==
  note: Entradas
  note: Controle de Atitude
  note: Saídas
  note: Resultados
  q_erro : Inport
  omega_rel : Inport  Port=2
  Demux : Demux
  Demux1 : Demux  Outputs=3
  Gain1 : Gain  Gain=-1
  Kd1 : Gain  Gain=[AttKd_x AttKd_y AttKd_z]'
  Kp1 : Gain  Gain=[AttKp_x AttKp_y AttKp_z]'
  Mux : Mux  Inputs=3
  Sum3 : Sum  Inputs=|++
  Terminator : Terminator
  Unit Delay : UnitDelay  SampleTime=-1  HasFrameUpgradeWarning=on
  Unit Delay1 : UnitDelay  SampleTime=-1  HasFrameUpgradeWarning=on
  Vector Concatenate1 : Concatenate  NumInputs=3  Mode=Multidimensional array
  Mts : Outport
  wires:
  [q_erro] -> Demux/1
  Mux/1 -> Kp1/1
  Demux/1 -> Mux/1
  Demux/2 -> Mux/2
  Demux/3 -> Mux/3
  Demux/4 -> Terminator/1
  [omega_rel] -> Kd1/1
  Kd1/1 -> Sum3/2
  Sum3/1 -> Demux1/1
  Demux1/1 -> Vector Concatenate1/1
  Demux1/2 -> Vector Concatenate1/2
  Demux1/3 -> Vector Concatenate1/3
  q_erro/1 -> Unit Delay/1
  omega_rel/1 -> Unit Delay1/1
  [Mts] -> Mts/1
  Vector Concatenate1/1 -> Gain1/1
  Gain1/1 -> [Mts]
  Kp1/1 -> Sum3/1
  Unit Delay/1 -> [q_erro]
  Unit Delay1/1 -> [omega_rel]

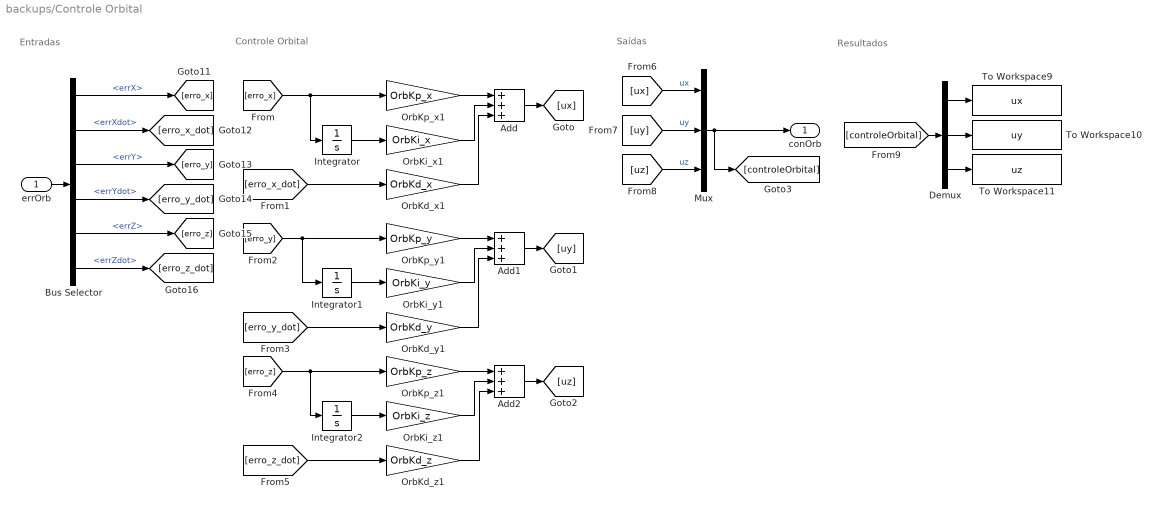
== system backups/Controle Orbital ==
  note: Entradas
  note: Controle Orbital
  note: Saídas
  note: Resultados
  errOrb : Inport
  Add : Sum  Inputs=+++
  Add1 : Sum  Inputs=+++
  Add2 : Sum  Inputs=+++
  Bus Selector : BusSelector  OutputSignals=errX,errXdot,errY,errYdot,errZ,errZdot
  Demux : Demux  Outputs=3
  Integrator : Integrator
  Integrator1 : Integrator
  Integrator2 : Integrator
  Mux : Mux  Inputs=3
  OrbKd_x1 : Gain  Gain=OrbKd_x
  OrbKd_y1 : Gain  Gain=OrbKd_y
  OrbKd_z1 : Gain  Gain=OrbKd_z
  OrbKi_x1 : Gain  Gain=OrbKi_x
  OrbKi_y1 : Gain  Gain=OrbKi_y
  OrbKi_z1 : Gain  Gain=OrbKi_z
  OrbKp_x1 : Gain  Gain=OrbKp_x
  OrbKp_y1 : Gain  Gain=OrbKp_y
  OrbKp_z1 : Gain  Gain=OrbKp_z
  To Workspace10 : ToWorkspace  VariableName=uy  SampleTime=-1
      settings: Save2DSignal=2-D array (concatenate along first dimension)
  To Workspace11 : ToWorkspace  VariableName=uz  SampleTime=-1
      settings: Save2DSignal=2-D array (concatenate along first dimension)
  To Workspace9 : ToWorkspace  VariableName=ux  SampleTime=-1
      settings: Save2DSignal=2-D array (concatenate along first dimension)
  conOrb : Outport
  wires:
  Add/1 -> [ux]
  Add1/1 -> [uy]
  Add2/1 -> [uz]
  Bus Selector/6 -> [erro_z_dot]  "<errZdot>"
  Bus Selector/4 -> [erro_y_dot]  "<errYdot>"
  Bus Selector/3 -> [erro_y]  "<errY>"
  Bus Selector/1 -> [erro_x]  "<errX>"
  Bus Selector/5 -> [erro_z]  "<errZ>"
  Bus Selector/2 -> [erro_x_dot]  "<errXdot>"
  errOrb/1 -> Bus Selector/1
  [ux] -> Mux/1  "ux"
  [uy] -> Mux/2  "uy"
  [uz] -> Mux/3  "uz"
  [erro_x_dot] -> OrbKd_x1/1
  Integrator1/1 -> OrbKi_y1/1
  Integrator2/1 -> OrbKi_z1/1
  [erro_y] -> OrbKp_y1/1, Integrator1/1
  OrbKi_z1/1 -> Add2/2
  OrbKi_x1/1 -> Add/2
  OrbKp_x1/1 -> Add/1
  OrbKd_x1/1 -> Add/3
  [erro_x] -> OrbKp_x1/1, Integrator/1
  OrbKi_y1/1 -> Add1/2
  OrbKp_y1/1 -> Add1/1
  Integrator/1 -> OrbKi_x1/1
  OrbKd_y1/1 -> Add1/3
  [erro_z_dot] -> OrbKd_z1/1
  OrbKd_z1/1 -> Add2/3
  [erro_y_dot] -> OrbKd_y1/1
  [erro_z] -> OrbKp_z1/1, Integrator2/1
  OrbKp_z1/1 -> Add2/1
  Mux/1 -> conOrb/1, [controleOrbital]
  Demux/3 -> To Workspace11/1
  [controleOrbital] -> Demux/1
  Demux/1 -> To Workspace9/1
  Demux/2 -> To Workspace10/1

== system backups/Controle Orbital1 ==
  note: Entradas
  note: Controle Orbital
  note: Saídas
  note: Resultados
  errOrb : Inport
  Add : Sum  Inputs=+++
  Add1 : Sum  Inputs=+++
  Add2 : Sum  Inputs=+++
  Bus Selector : BusSelector  OutputSignals=errX,errXdot,errY,errYdot,errZ,errZdot
  Integrator : Integrator
  Integrator1 : Integrator
  Integrator2 : Integrator
  Mux : Mux  Inputs=3
  OrbKd_x1 : Gain  Gain=OrbKd_x
  OrbKd_y1 : Gain  Gain=OrbKd_y
  OrbKd_z1 : Gain  Gain=OrbKd_z
  OrbKi_x1 : Gain  Gain=OrbKi_x
  OrbKi_y1 : Gain  Gain=OrbKi_y
  OrbKi_z1 : Gain  Gain=OrbKi_z
  OrbKp_x1 : Gain  Gain=OrbKp_x
  OrbKp_y1 : Gain  Gain=OrbKp_y
  OrbKp_z1 : Gain  Gain=OrbKp_z
  conOrb : Outport
  wires:
  Add/1 -> [ux]
  Add1/1 -> [uy]
  Add2/1 -> [uz]
  Bus Selector/6 -> [erro_z_dot]  "<errZdot>"
  Bus Selector/4 -> [erro_y_dot]  "<errYdot>"
  Bus Selector/3 -> [erro_y]  "<errY>"
  Bus Selector/1 -> [erro_x]  "<errX>"
  Bus Selector/5 -> [erro_z]  "<errZ>"
  Bus Selector/2 -> [erro_x_dot]  "<errXdot>"
  errOrb/1 -> Bus Selector/1
  [ux] -> Mux/1  "ux"
  [uy] -> Mux/2  "uy"
  [uz] -> Mux/3  "uz"
  [erro_x_dot] -> OrbKd_x1/1
  Integrator1/1 -> OrbKi_y1/1
  Integrator2/1 -> OrbKi_z1/1
  [erro_y] -> OrbKp_y1/1, Integrator1/1
  OrbKi_z1/1 -> Add2/2
  OrbKi_x1/1 -> Add/2
  OrbKp_x1/1 -> Add/1
  OrbKd_x1/1 -> Add/3
  [erro_x] -> OrbKp_x1/1, Integrator/1
  OrbKi_y1/1 -> Add1/2
  OrbKp_y1/1 -> Add1/1
  Integrator/1 -> OrbKi_x1/1
  OrbKd_y1/1 -> Add1/3
  [erro_z_dot] -> OrbKd_z1/1
  OrbKd_z1/1 -> Add2/3
  [erro_y_dot] -> OrbKd_y1/1
  [erro_z] -> OrbKp_z1/1, Integrator2/1
  OrbKp_z1/1 -> Add2/1
  Mux/1 -> conOrb/1, [controleOrbital]

== system backups/ControleAtitude1 ==
  note: Entradas
  note: Planta
  note: Saídas
  q_erro : Inport
  omega_rel : Inport  Port=2
  Demux : Demux
  Demux1 : Demux  Outputs=3
  Gain1 : Gain  Gain=-1
  Kd1 : Gain  Gain=[AttKd_x AttKd_y AttKd_z]'
  Kp1 : Gain  Gain=[AttKp_x AttKp_y AttKp_z]'
  Mux : Mux  Inputs=3
  Sum3 : Sum  Inputs=|++
  Terminator : Terminator
  Vector Concatenate1 : Concatenate  NumInputs=3  Mode=Multidimensional array
  Mts : Outport
  wires:
  [q_erro] -> Demux/1
  Mux/1 -> Kp1/1
  Demux/1 -> Mux/1
  Demux/2 -> Mux/2
  Demux/3 -> Mux/3
  Demux/4 -> Terminator/1
  [omega_rel] -> Kd1/1
  Kd1/1 -> Sum3/2
  Sum3/1 -> Demux1/1
  Demux1/1 -> Vector Concatenate1/1
  Demux1/2 -> Vector Concatenate1/2
  Demux1/3 -> Vector Concatenate1/3
  q_erro/1 -> [q_erro]
  omega_rel/1 -> [omega_rel]
  [Mts] -> Mts/1
  Vector Concatenate1/1 -> Gain1/1
  Gain1/1 -> [Mts]
  Kp1/1 -> Sum3/1

== system backups/Dinâmica Cinemática Atitude ==
  note: Dinâmica e Cinemática de Atitude
  note: Saídas
  note: Entradas
  note: Resultados
  dinCinOrb : Inport
  Mts : Inport  Port=2
  Bus Creator : BusCreator  Inputs=3
  Bus Selector : BusSelector  OutputSignals=omega_x,omega_y,omega_z,omega_x_dot,omega_y_dot,omega_z_dot
  Bus Selector4 : BusSelector  OutputSignals=phi,theta,psi
  DinamicaCinematicaAtitude : ModelReference  ModelNameDialog=DinamicaCinematicaControleAtitude  ModelReferenceVersion=3.14
  MATLAB Function : MATLAB Function  TreatAsAtomicUnit=on
  To Workspace15 : ToWorkspace  VariableName=phi  SampleTime=-1
      settings: Save2DSignal=2-D array (concatenate along first dimension)
  To Workspace16 : ToWorkspace  VariableName=theta  SampleTime=-1
      settings: Save2DSignal=2-D array (concatenate along first dimension)
  To Workspace17 : ToWorkspace  VariableName=psi  SampleTime=-1
      settings: Save2DSignal=2-D array (concatenate along first dimension)
  Vector Concatenate : Concatenate  NumInputs=3  Mode=Multidimensional array
  Vector Concatenate1 : Concatenate  NumInputs=3  Mode=Multidimensional array
  q_rel : Outport
  A_q : Outport  Port=2
  omega_rel : Outport  Port=3
  wires:
  DinamicaCinematicaAtitude/1 -> [q_rel]
  DinamicaCinematicaAtitude/2 -> [A_q]
  [q_rel] -> q_rel/1
  dinCinOrb/1 -> Bus Selector/1
  [omega_i] -> DinamicaCinematicaAtitude/2
  [omega_i_dot] -> DinamicaCinematicaAtitude/3
  [Mts] -> DinamicaCinematicaAtitude/1
  Bus Selector/1 -> Vector Concatenate1/1  "<omega_x>"
  Bus Selector/3 -> Vector Concatenate1/3  "<omega_z>"
  Bus Selector/2 -> Vector Concatenate1/2  "<omega_y>"
  Vector Concatenate1/1 -> [omega_i]
  Bus Selector/4 -> Vector Concatenate/1  "<omega_x_dot>"
  Bus Selector/5 -> Vector Concatenate/2  "<omega_y_dot>"
  Bus Selector/6 -> Vector Concatenate/3  "<omega_z_dot>"
  Vector Concatenate/1 -> [omega_i_dot]
  DinamicaCinematicaAtitude/3 -> [omega_rel]
  Mts/1 -> [Mts]
  [q_rel] -> MATLAB Function/1(u)
  MATLAB Function/1(phi) -> Bus Creator/1
  MATLAB Function/2(theta) -> Bus Creator/2
  MATLAB Function/3(psi) -> Bus Creator/3
  [A_q] -> A_q/1
  [omega_rel] -> omega_rel/1
  Bus Selector4/2 -> To Workspace16/1  "<theta>"
  Bus Selector4/1 -> To Workspace15/1  "<phi>"
  [atitude] -> Bus Selector4/1
  Bus Selector4/3 -> To Workspace17/1  "<psi>"
  Bus Creator/1 -> [atitude]

== system backups/Dinâmica Cinemática Atitude1 ==
  note: Dinâmica e Cinemática de Atitude
  note: Saídas
  note: Entradas
  note: Resultados
  dinCinOrb : Inport
  Mts : Inport  Port=2
  Bus Creator : BusCreator  Inputs=3
  Bus Selector : BusSelector  OutputSignals=omega_x,omega_y,omega_z,omega_x_dot,omega_y_dot,omega_z_dot
  Bus Selector4 : BusSelector  OutputSignals=phi,theta,psi
  DinamicaCinematicaAtitude : ModelReference  ModelNameDialog=DinamicaCinematicaControleAtitude  ModelReferenceVersion=3.14
  MATLAB Function : MATLAB Function  TreatAsAtomicUnit=on
  To Workspace15 : ToWorkspace  VariableName=phi  SampleTime=-1
      settings: Save2DSignal=2-D array (concatenate along first dimension)
  To Workspace16 : ToWorkspace  VariableName=theta  SampleTime=-1
      settings: Save2DSignal=2-D array (concatenate along first dimension)
  To Workspace17 : ToWorkspace  VariableName=psi  SampleTime=-1
      settings: Save2DSignal=2-D array (concatenate along first dimension)
  Vector Concatenate : Concatenate  NumInputs=3  Mode=Multidimensional array
  Vector Concatenate1 : Concatenate  NumInputs=3  Mode=Multidimensional array
  q_rel : Outport
  A_q : Outport  Port=2
  omega_rel : Outport  Port=3
  wires:
  DinamicaCinematicaAtitude/1 -> [q_rel]
  DinamicaCinematicaAtitude/2 -> [A_q]
  [q_rel] -> q_rel/1
  dinCinOrb/1 -> Bus Selector/1
  [omega_i] -> DinamicaCinematicaAtitude/2
  [omega_i_dot] -> DinamicaCinematicaAtitude/3
  [Mts] -> DinamicaCinematicaAtitude/1
  Bus Selector/1 -> Vector Concatenate1/1  "<omega_x>"
  Bus Selector/3 -> Vector Concatenate1/3  "<omega_z>"
  Bus Selector/2 -> Vector Concatenate1/2  "<omega_y>"
  Vector Concatenate1/1 -> [omega_i]
  Bus Selector/4 -> Vector Concatenate/1  "<omega_x_dot>"
  Bus Selector/5 -> Vector Concatenate/2  "<omega_y_dot>"
  Bus Selector/6 -> Vector Concatenate/3  "<omega_z_dot>"
  Vector Concatenate/1 -> [omega_i_dot]
  DinamicaCinematicaAtitude/3 -> [omega_rel]
  Mts/1 -> [Mts]
  [q_rel] -> MATLAB Function/1(u)
  MATLAB Function/1(phi) -> Bus Creator/1
  MATLAB Function/2(theta) -> Bus Creator/2
  MATLAB Function/3(psi) -> Bus Creator/3
  [A_q] -> A_q/1
  [omega_rel] -> omega_rel/1
  Bus Selector4/2 -> To Workspace16/1  "<theta>"
  Bus Selector4/1 -> To Workspace15/1  "<phi>"
  [atitude] -> Bus Selector4/1
  Bus Selector4/3 -> To Workspace17/1  "<psi>"
  Bus Creator/1 -> [atitude]

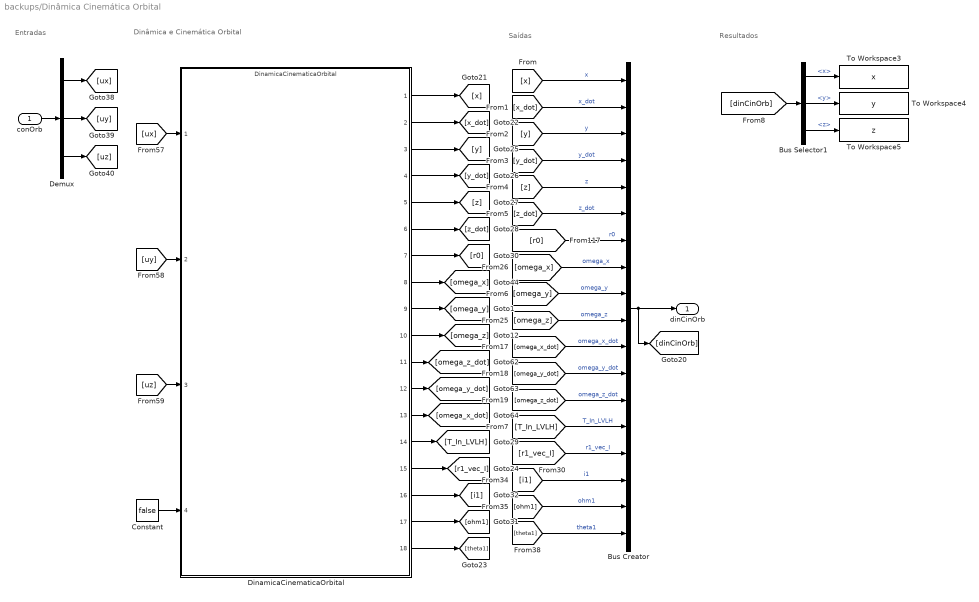
== system backups/Dinâmica Cinemática Orbital ==
  note: Entradas
  note: Saídas
  note: Dinâmica e Cinemática Orbital
  note: Resultados
  conOrb : Inport  OutDataTypeStr=double
  Bus Creator : BusCreator  Inputs=18
  Bus Selector1 : BusSelector  OutputSignals=x,y,z
  Constant : Constant  Value=false
  Demux : Demux  Outputs=3
  DinamicaCinematicaOrbital : ModelReference  ModelNameDialog=DinamicaCinematicaOrbital  ModelReferenceVersion=5.18
  To Workspace3 : ToWorkspace  VariableName=x  SampleTime=-1
      settings: Save2DSignal=2-D array (concatenate along first dimension)
  To Workspace4 : ToWorkspace  VariableName=y  SampleTime=-1
      settings: Save2DSignal=2-D array (concatenate along first dimension)
  To Workspace5 : ToWorkspace  VariableName=z  SampleTime=-1
      settings: Save2DSignal=2-D array (concatenate along first dimension)
  dinCinOrb : Outport
  wires:
  conOrb/1 -> Demux/1
  Demux/1 -> [ux]
  Demux/2 -> [uy]
  Demux/3 -> [uz]
  [ux] -> DinamicaCinematicaOrbital/1
  [uy] -> DinamicaCinematicaOrbital/2
  [uz] -> DinamicaCinematicaOrbital/3
  Constant/1 -> DinamicaCinematicaOrbital/4
  Bus Creator/1 -> dinCinOrb/1, [dinCinOrb]
  Bus Selector1/1 -> To Workspace3/1  "<x>"
  Bus Selector1/2 -> To Workspace4/1  "<y>"
  Bus Selector1/3 -> To Workspace5/1  "<z>"
  [dinCinOrb] -> Bus Selector1/1
  DinamicaCinematicaOrbital/2 -> [x_dot]
  DinamicaCinematicaOrbital/5 -> [z]
  DinamicaCinematicaOrbital/4 -> [y_dot]
  DinamicaCinematicaOrbital/6 -> [z_dot]
  DinamicaCinematicaOrbital/7 -> [r0]
  DinamicaCinematicaOrbital/3 -> [y]
  DinamicaCinematicaOrbital/1 -> [x]
  DinamicaCinematicaOrbital/8 -> [omega_x]
  DinamicaCinematicaOrbital/10 -> [omega_z]
  DinamicaCinematicaOrbital/11 -> [omega_z_dot]
  DinamicaCinematicaOrbital/12 -> [omega_y_dot]
  DinamicaCinematicaOrbital/13 -> [omega_x_dot]
  DinamicaCinematicaOrbital/14 -> [T_In_LVLH]
  DinamicaCinematicaOrbital/15 -> [r1_vec_I]
  DinamicaCinematicaOrbital/16 -> [i1]
  DinamicaCinematicaOrbital/17 -> [ohm1]
  DinamicaCinematicaOrbital/18 -> [theta1]
  DinamicaCinematicaOrbital/9 -> [omega_y]
  [theta1] -> Bus Creator/18  "theta1"
  [ohm1] -> Bus Creator/17  "ohm1"
  [i1] -> Bus Creator/16  "i1"
  [r1_vec_I] -> Bus Creator/15  "r1_vec_I"
  [T_In_LVLH] -> Bus Creator/14  "T_In_LVLH"
  [omega_z_dot] -> Bus Creator/13  "omega_z_dot"
  [omega_y_dot] -> Bus Creator/12  "omega_y_dot"
  [omega_x_dot] -> Bus Creator/11  "omega_x_dot"
  [omega_z] -> Bus Creator/10  "omega_z"
  [omega_y] -> Bus Creator/9  "omega_y"
  [omega_x] -> Bus Creator/8  "omega_x"
  [r0] -> Bus Creator/7  "r0"
  [z_dot] -> Bus Creator/6  "z_dot"
  [z] -> Bus Creator/5  "z"
  [y_dot] -> Bus Creator/4  "y_dot"
  [y] -> Bus Creator/3  "y"
  [x_dot] -> Bus Creator/2  "x_dot"
  [x] -> Bus Creator/1  "x"

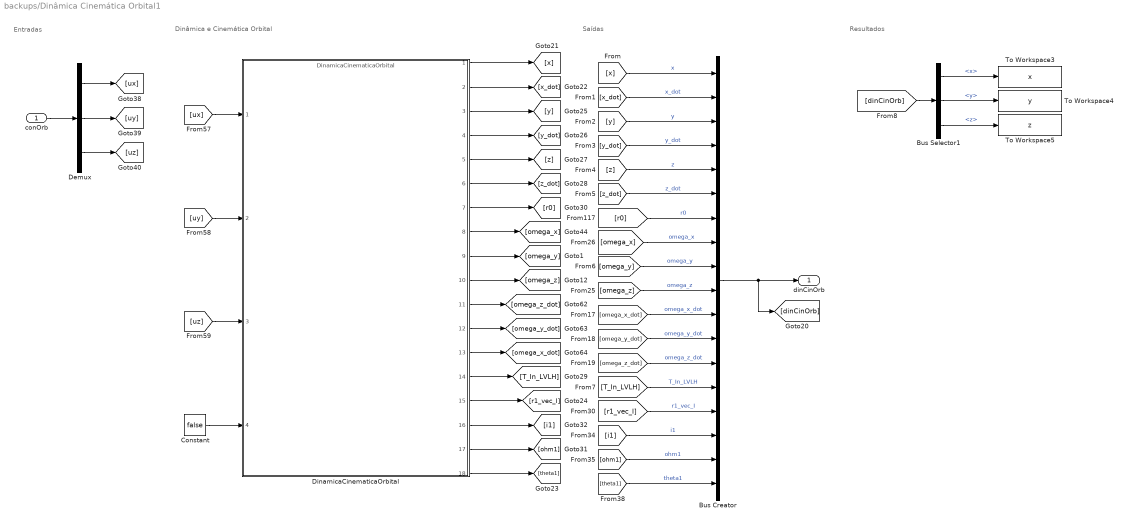
== system backups/Dinâmica Cinemática Orbital1 ==
  note: Entradas
  note: Saídas
  note: Dinâmica e Cinemática Orbital
  note: Resultados
  conOrb : Inport  OutDataTypeStr=double
  Bus Creator : BusCreator  Inputs=18
  Bus Selector1 : BusSelector  OutputSignals=x,y,z
  Constant : Constant  Value=false
  Demux : Demux  Outputs=3
  DinamicaCinematicaOrbital : ModelReference  ModelNameDialog=DinamicaCinematicaOrbital  ModelReferenceVersion=5.18
  To Workspace3 : ToWorkspace  VariableName=x  SampleTime=-1
      settings: Save2DSignal=2-D array (concatenate along first dimension)
  To Workspace4 : ToWorkspace  VariableName=y  SampleTime=-1
      settings: Save2DSignal=2-D array (concatenate along first dimension)
  To Workspace5 : ToWorkspace  VariableName=z  SampleTime=-1
      settings: Save2DSignal=2-D array (concatenate along first dimension)
  dinCinOrb : Outport
  wires:
  conOrb/1 -> Demux/1
  Demux/1 -> [ux]
  Demux/2 -> [uy]
  Demux/3 -> [uz]
  [ux] -> DinamicaCinematicaOrbital/1
  [uy] -> DinamicaCinematicaOrbital/2
  [uz] -> DinamicaCinematicaOrbital/3
  Constant/1 -> DinamicaCinematicaOrbital/4
  Bus Creator/1 -> dinCinOrb/1, [dinCinOrb]
  Bus Selector1/1 -> To Workspace3/1  "<x>"
  Bus Selector1/2 -> To Workspace4/1  "<y>"
  Bus Selector1/3 -> To Workspace5/1  "<z>"
  [dinCinOrb] -> Bus Selector1/1
  DinamicaCinematicaOrbital/2 -> [x_dot]
  DinamicaCinematicaOrbital/5 -> [z]
  DinamicaCinematicaOrbital/4 -> [y_dot]
  DinamicaCinematicaOrbital/6 -> [z_dot]
  DinamicaCinematicaOrbital/7 -> [r0]
  DinamicaCinematicaOrbital/3 -> [y]
  DinamicaCinematicaOrbital/1 -> [x]
  DinamicaCinematicaOrbital/8 -> [omega_x]
  DinamicaCinematicaOrbital/10 -> [omega_z]
  DinamicaCinematicaOrbital/11 -> [omega_z_dot]
  DinamicaCinematicaOrbital/12 -> [omega_y_dot]
  DinamicaCinematicaOrbital/13 -> [omega_x_dot]
  DinamicaCinematicaOrbital/14 -> [T_In_LVLH]
  DinamicaCinematicaOrbital/15 -> [r1_vec_I]
  DinamicaCinematicaOrbital/16 -> [i1]
  DinamicaCinematicaOrbital/17 -> [ohm1]
  DinamicaCinematicaOrbital/18 -> [theta1]
  DinamicaCinematicaOrbital/9 -> [omega_y]
  [theta1] -> Bus Creator/18  "theta1"
  [ohm1] -> Bus Creator/17  "ohm1"
  [i1] -> Bus Creator/16  "i1"
  [r1_vec_I] -> Bus Creator/15  "r1_vec_I"
  [T_In_LVLH] -> Bus Creator/14  "T_In_LVLH"
  [omega_z_dot] -> Bus Creator/13  "omega_z_dot"
  [omega_y_dot] -> Bus Creator/12  "omega_y_dot"
  [omega_x_dot] -> Bus Creator/11  "omega_x_dot"
  [omega_z] -> Bus Creator/10  "omega_z"
  [omega_y] -> Bus Creator/9  "omega_y"
  [omega_x] -> Bus Creator/8  "omega_x"
  [r0] -> Bus Creator/7  "r0"
  [z_dot] -> Bus Creator/6  "z_dot"
  [z] -> Bus Creator/5  "z"
  [y_dot] -> Bus Creator/4  "y_dot"
  [y] -> Bus Creator/3  "y"
  [x_dot] -> Bus Creator/2  "x_dot"
  [x] -> Bus Creator/1  "x"
